simulink model "Catmull_Rom"  (R2023b)
settings: Solver=FixedStepDiscrete  StartTime=0.0  StopTime=3.999  FixedStep=0.02  RelTol=1e-3
StopFcn:
  | Catmull_Rom_Plotting
undefined symbols (not defined in the file or in its folder): Spline_Num_Poses_auto, Spline_Ref_Poses_auto
libraries: SignalEditorBlockLib x1
settings Model: Creator=FIRSTMentor  LastModifiedBy=ander
settings OptimizationCC: DefaultParameterBehavior=Inlined  EnhancedBackFolding=on  PassReuseOutputArgsAs=Individual arguments  ZeroExternalMemoryAtStartup=off  ZeroInternalMemoryAtStartup=off  OptimizeBlockOrder=speed  DifferentSizesBufferReuse=on  OptimizationCustomize=off  EfficientTunableParamExpr=on
settings DebuggingCC: ParameterTunabilityLossMsg=error
settings SFSimCC: MATLABDynamicMemAlloc=off
settings RTWCC: Description=Embedded Coder  SystemTargetFile=ert.tlc  GenCodeOnly=on  TemplateMakefile=ert_default_tmf  Toolchain=Microsoft Visual C++ 2022 v17.0 | CMake/nmake (64-bit Windows)  BuildConfiguration=Release
settings CodeAppCC: ForceParamTrailComments=on  IgnoreCustomStorageClasses=off  OperatorAnnotations=on  SimulinkDataObjDesc=on  SFDataObjDesc=on  InsertBlockDesc=on
settings ERTTargetCC: TargetLangStandard=C99 (ISO)  GenerateSampleERTMain=on  InlinedParameterPlacement=NonHierarchical  ERTCustomFileTemplate=example_file_process.tlc

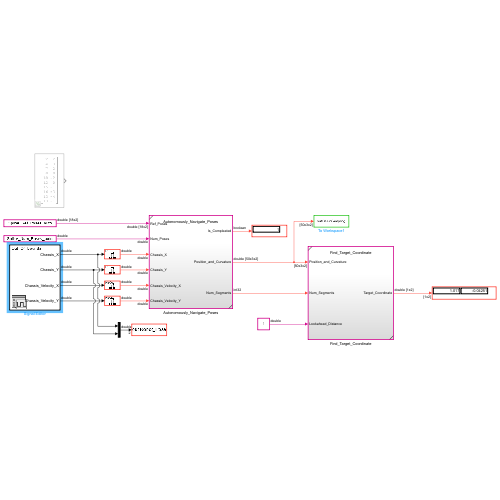
[thumbnail: Simulink's stored preview of the top-level diagram]
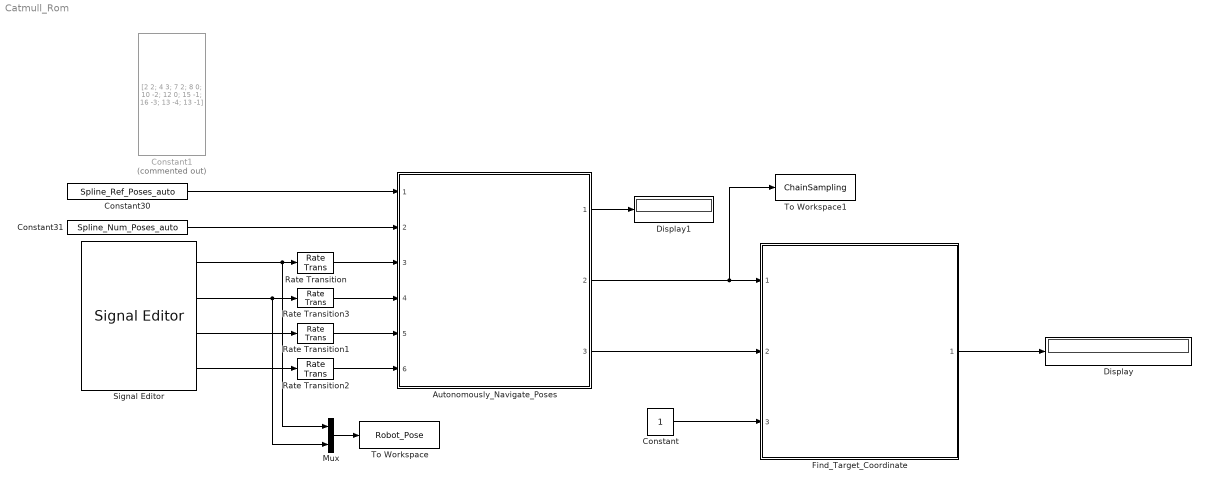
== system Catmull_Rom ==
  Autonomously_Navigate_Poses : Subsystem  ReferencedSubsystem=Autonomously_Navigate_Poses
  Constant : Constant
  Constant1 : Constant  Commented=on  Value=[2 2; 4 3; 7 2; 8 0; 10 -2; 12 0; 15 -1; 16 -3; 13 -4; 13 -1]
  Constant30 : Constant  Value=Spline_Ref_Poses_auto
  Constant31 : Constant  Value=Spline_Num_Poses_auto  OutDataTypeStr=double
  Display : Display
  Display1 : Display
  Find_Target_Coordinate : Subsystem  ReferencedSubsystem=Find_Target_Coordinate
  Mux : Mux  Inputs=2
  Rate Transition{,1..3} (4 alike) : RateTransition  OutPortSampleTime=t_sample
  Signal Editor : SignalEditorBlockLib/Signal Editor  FileName=Catmull_Rom_Path_Test_Cases.mat  ActiveScenario=Out_Of_Bounds  ActiveSignal=Chassis_X  IsBus=off  OutputBusObjectStr=Bus: BusObject  SampleTime=0  Interpolate=off  ZeroCross=off  OutputAfterFinalValue=Setting to zero  Unit=inherit  PreserveSignalName=on  ApplySigPropsToAllScenarios=on  ApplySigPropsToAllSignals=off
  To Workspace : ToWorkspace  VariableName=Robot_Pose  SampleTime=-1
      settings: Save2DSignal=2-D array (concatenate along first dimension)
  To Workspace1 : ToWorkspace  VariableName=ChainSampling  SaveFormat=Structure  SampleTime=20
  wires:
  Constant30/1 -> Autonomously_Navigate_Poses/1
  Constant31/1 -> Autonomously_Navigate_Poses/2
  Signal Editor/1 -> Mux/1, Rate Transition/1
  Signal Editor/2 -> Rate Transition3/1, Mux/2
  Signal Editor/3 -> Rate Transition1/1
  Signal Editor/4 -> Rate Transition2/1
  Rate Transition/1 -> Autonomously_Navigate_Poses/3
  Rate Transition1/1 -> Autonomously_Navigate_Poses/5
  Rate Transition2/1 -> Autonomously_Navigate_Poses/6
  Rate Transition3/1 -> Autonomously_Navigate_Poses/4
  Mux/1 -> To Workspace/1
  Find_Target_Coordinate/1 -> Display/1
  Constant/1 -> Find_Target_Coordinate/3
  Autonomously_Navigate_Poses/2 -> To Workspace1/1, Find_Target_Coordinate/1
  Autonomously_Navigate_Poses/3 -> Find_Target_Coordinate/2
  Autonomously_Navigate_Poses/1 -> Display1/1
